simulink model "phi1_helicopter_breach"  (R2017a)
settings: Solver=ode45  StartTime=0.0  StopTime=tspan(end)  RelTol=1e-3  EnableMultiTasking=on
model workspace (MAT data in the model file):
  Con = 0
  Gai = 0
undefined symbols (not defined in the file or in its folder): a, i, K
settings Model: Creator=alex  LastModifiedBy=nikhil
settings DataIOCC: ExternalInput=[t__, u__]  LoadExternalInput=on  SaveFormat=StructureWithTime  ReturnWorkspaceOutputs=on
settings OptimizationCC: LifeSpan=inf
settings DebuggingCC: SFUnexpectedBacktrackingDiag=warning  SFNoUnconditionalDefaultTransitionDiag=warning  SFExecutionAtInitializationDiag=none
settings HardwareCC: ProdBitPerPointer=32  ProdBitPerSizeT=32  ProdBitPerPtrDiffT=32  ProdLargestAtomicFloat=None  ProdIntDivRoundTo=Undefined  ProdEndianess=Unspecified  ProdWordSize=32  ProdHWDeviceType=32-bit Generic
settings ModelReferenceCC: PropagateSignalLabelsOutOfModel=off
settings GRTTargetCC: TargetLangStandard=C89/C90 (ANSI)  GeneratePreprocessorConditionals=Disable all
settings ConfigComp: CovMetricSettings=dw  CovHtmlReporting=on  CovSaveCumulativeToWorkspaceVar=on  CovSaveSingleToWorkspaceVar=on  CovExternalEMLEnable=off  CovSFcnEnable=off

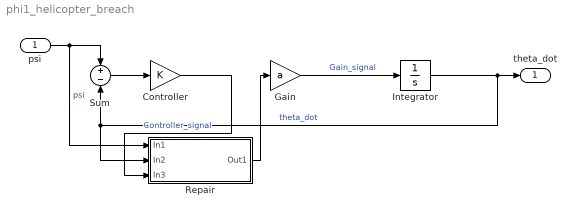
== system phi1_helicopter_breach ==
  psi : Inport
  "Controller " : Gain  Gain=K
  Gain : Gain  Gain=a
  Integrator : Integrator  InitialCondition=i
  Repair : Subsystem
  Sum : Sum  Inputs=+-
  theta_dot : Outport
  wires:
  Gain/1 -> Integrator/1  "Gain_signal"
  Integrator/1 -> theta_dot/1, Repair/2(In2), Sum/2  "theta_dot"
  "Controller "/1 -> Repair/3(In3)  "Controller_signal"
  psi/1 -> Repair/1(In1), Sum/1  "psi"
  Sum/1 -> "Controller "/1
  Repair/1(Out1) -> Gain/1

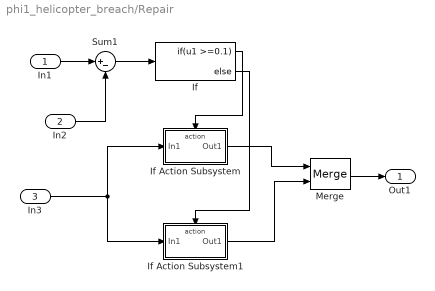
== system phi1_helicopter_breach/Repair ==
  In1 : Inport
  In2 : Inport  Port=2
  In3 : Inport  Port=3
  If : If  IfExpression=u1 >=0.1
  If Action Subsystem : Subsystem  TreatAsAtomicUnit=on
  If Action Subsystem1 : Subsystem  TreatAsAtomicUnit=on
  Merge : Merge
  Sum1 : Sum  Inputs=|+-
  Out1 : Outport
  wires:
  If Action Subsystem/1(Out1) -> Merge/1
  If/2 -> If Action Subsystem1/Action
  If/1 -> If Action Subsystem/Action
  Sum1/1 -> If/1
  If Action Subsystem1/1(Out1) -> Merge/2
  In1/1 -> Sum1/1
  In2/1 -> Sum1/2
  Merge/1 -> Out1/1
  In3/1 -> If Action Subsystem1/1(In1), If Action Subsystem/1(In1)

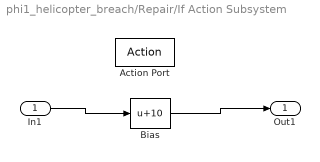
== system phi1_helicopter_breach/Repair/If Action Subsystem ==
  In1 : Inport
  Action Port : ActionPort  ActionType=then
  Bias : Bias  Bias=10
  Out1 : Outport
  wires:
  In1/1 -> Bias/1
  Bias/1 -> Out1/1

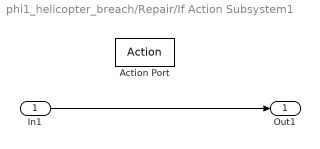
== system phi1_helicopter_breach/Repair/If Action Subsystem1 ==
  In1 : Inport
  Action Port : ActionPort  ActionType=else
  Out1 : Outport
  wires:
  In1/1 -> Out1/1
